simulink model "lqrSimulink"  (R2023a)
settings: Solver=VariableStepAuto  StartTime=0.0  StopTime=10.0  RelTol=1e-3
settings Model: Creator=belov  LastModifiedBy=belov

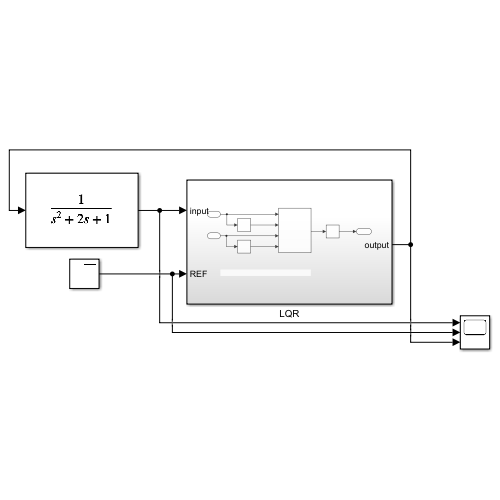
[thumbnail: Simulink's stored preview of the top-level diagram]
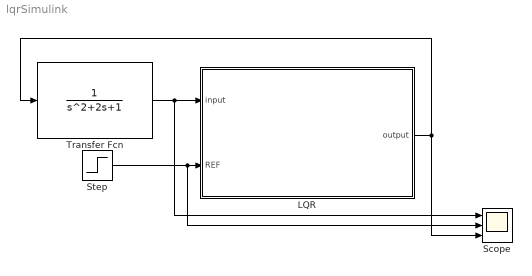
== system lqrSimulink ==
  LQR : Subsystem
  Scope : Scope  NumInputPorts=3
  Step : Step  SampleTime=0.01
  Transfer Fcn : TransferFcn
  wires:
  Transfer Fcn/1 -> Scope/1, LQR/1(input)
  LQR/1(output) -> Transfer Fcn/1, Scope/3
  Step/1 -> Scope/2, LQR/2(REF)

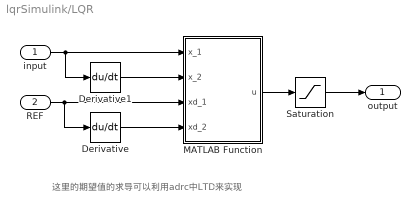
== system lqrSimulink/LQR ==
  note: 这里的期望值的求导可以利用adrc中LTD来实现
  input : Inport
  REF : Inport  Port=2
  Derivative : Derivative
  Derivative1 : Derivative
  MATLAB Function : MATLAB Function  TreatAsAtomicUnit=on
  Saturation : Saturate  UpperLimit=5  LowerLimit=-5
  output : Outport
  wires:
  input/1 -> MATLAB Function/1(x_1), Derivative1/1
  MATLAB Function/1(u) -> Saturation/1
  REF/1 -> MATLAB Function/3(xd_1), Derivative/1
  Derivative/1 -> MATLAB Function/4(xd_2)
  Derivative1/1 -> MATLAB Function/2(x_2)
  Saturation/1 -> output/1

== matlab function lqrSimulink/LQR/MATLAB Function ==
  settings: updateMethod=DISCRETE
  data: x_1 input; u output; x_2 input; xd_1 input; xd_2 input
function u = fcn(x_1, x_2, xd_1, xd_2)

X = [x_1 - xd_1; x_2 - xd_2];
F = [9.0499 9.0499];
u =  -F * X;

end
